simulink library "NCS_Library"  (R2019a)
settings: Solver=VariableStepAuto  StartTime=0.0  StopTime=10.0  RelTol=1e-3
values from neighbouring files (symbols this model uses):
  A = 10    [Parameter.m]
  band = 100000000    [Parameter.m]
  BER = 0    [Parameter.m]
  c = 5000000    [Parameter.m]
  c1 = 4.33    [Parameter.m]
  c2 = 3.16    [Parameter.m]
  CAN2EthernetDelay = 0.000    (= 0)    [Parameter.m]
  cR = 1.5*10^-3    (= 0.0015)    [Parameter.m]
  cw = (cwE * 2 + cwM * (nW_ges-2))/nW_ges    (= 0.1475)    [Parameter.m]
  cwE = 0.35    [Parameter.m]
  cwM = 0.08    [Parameter.m]
  Cycle_Controller = 0    [Parameter.m]
  CyclePLC = 24/1000    (= 0.024)    [Parameter.m]
  d = 800000    [Parameter.m]
  Dr = 0.92    [Parameter.m]
  Ethernet2CANDelay = 0.005    [Parameter.m]
  F_konst = 70892    [Parameter.m]
  FA = 100000    [Parameter.m]
  FB_WB_max = 10000    [Parameter.m]
  FBel_an = iG*nG*F_KZmax*nBan*R_mR/(Dr/2)    (= 28197.4297239)    [Parameter.m]
  FBel_frei = iG*nG*F_KZmax*nBfrei*R_mW/(Dr/2)    (= 29270.6882948)    [Parameter.m]
  Fmaxdyn = 300000    [Parameter.m]
  g = 9.81    [Parameter.m]
  i = 0    [Parameter.m]
  J = 1/2*mA*(Dr/2)^2    (= 158.7)    [Parameter.m]
  k1 = 0.095    [Parameter.m]
  k2 = 9.26/3.6    (= 2.57222222222)    [Parameter.m]
  k3 = 4.63/3.6    (= 1.28611111111)    [Parameter.m]
  mges = 58000    [Parameter.m]
  mu = [mu1 mu2]    [Parameter.m]
  muBel1 = 0.42    [Parameter.m]
  muBel2 = 0.36    [Parameter.m]
  n = 0.001    [Parameter.m]
  n_Mg = 4    [Parameter.m]
  n_WB = 4    [Parameter.m]
  nA = 4    [Parameter.m]
  nBan = 2    [Parameter.m]
  nBfrei = 3    [Parameter.m]
  nM = 4    [Parameter.m]
  nW_an = 4    [Parameter.m]
  P_max = 8200000    [Parameter.m]
  Q = 10    [Parameter.m]
  r_reib = 600    [Parameter.m]
  rho = 1.08    [Parameter.m]
  rhoL = 1.225    [Parameter.m]
  Size = 8    [Parameter.m]
  slip = [s1 s2]    [Parameter.m]
  tol = 0.05    [Parameter.m]
  v00 = 100/3.6    (= 27.7777777778)    [Parameter.m]
  v_grenz = 60/3.6    (= 16.6666666667)    [Parameter.m]
  v_opt = 75/3.6    (= 20.8333333333)    [Parameter.m]
  W_opt = 0.5    [Parameter.m]
  WB = 1    [Parameter.m]
  y_opt = sqrt(W_opt)/((1+sqrt(W_opt))^2+W_opt)    [Parameter.m]
undefined symbols (not defined in the file or in its folder): BUSCapacity, CableLength, controlGate, D_dyn, D_mg, EnableBurst, EnableToF, entity, Entity_out, Gate, Gate_4, Gate_5, Gate_ACK, Gate_copy, Gate_RX, getData, gettime, I_dyn, I_mg, m, magnitude, P_dyn, P_mg, ReadAttributes, readdata, ReadData, ReadSize, sigbuilder_block, Timeout, ToB, ToF, v0, v_d, v_soll
libraries: simulink x176, $bdroot x102
(part 3 of 12)

== system NCS_Library/Plant (Train)/freier Wagen ==
  F_t : Inport
  F_vorne : Inport  Port=2
  F_hinten : Inport  Port=3
  fSt_WB : Inport  Port=4
  Add : Sum  Inputs=+-+--
  Bremskraft Schienenbremse : Subsystem
  Constant : Constant  Value=i
  Display : Display
  Display1 : Display
  Divide : Product  Inputs=*/
  Fahrwiderstand_Wagen : Subsystem
  Integrator : Integrator  InitialCondition=v0  LimitOutput=on  LowerSaturationLimit=tol  ShowSaturationPort=on
  Integrator1 : Integrator
  Scope : Scope
  Wagenmasse : Constant  Value=mges
  rho : Gain  Gain=rho
  v : Outport
  a : Outport  Port=2
  s : Outport  Port=3
  wires:
  rho/1 -> Divide/2
  Add/1 -> Divide/1
  Integrator1/1 -> s/1  "s"
  Constant/1 -> Fahrwiderstand_Wagen/1(Neigung in Promille)
  Wagenmasse/1 -> rho/1, Fahrwiderstand_Wagen/3(mges)
  F_vorne/1 -> Add/3
  Integrator/1 -> v/1, Bremskraft Schienenbremse/1(v), Fahrwiderstand_Wagen/2(v), Integrator1/1  "v"
  F_hinten/1 -> Add/4
  Divide/1 -> Integrator/1, a/1  "a"
  Integrator/2 -> Scope/1
  fSt_WB/1 -> Bremskraft Schienenbremse/2(fSt WB)
  F_t/1 -> Display/1, Add/1
  Bremskraft Schienenbremse/1(FB_frei) -> Add/2
  Fahrwiderstand_Wagen/1(Fw) -> Display1/1, Add/5

== system NCS_Library/Controller/Cookie/Braking Controller ==
  Fahrstufe : Inport
  Bremsstufe : Inport  Port=2
  Notbremse : Inport  Port=3
  v : Inport  Port=4
  Add : Sum
  Bremsen : Subsystem
  Compare To Constant : simulink/Logic and Bit Operations/Compare To Constant  relop===  const=3.0  OutDataTypeStr=boolean
  Compare To Constant1 : simulink/Logic and Bit Operations/Compare To Constant  relop===  const=4  OutDataTypeStr=boolean
  Constant : Constant  Value=v_soll
  Constant1 : Constant
  Demux : Demux  Outputs=3
  Display : Display
  Display1 : Display
  Leerlauf : Subsystem
  Logical Operator : Logic  Operator=OR  AllPortsSameDT=off  OutDataTypeStr=boolean
  Memory : Memory
  Multiport Switch : MultiPortSwitch  Inputs=4  DiagnosticForDefault=None
  Mux : Mux  Inputs=3
  Notbremsung : Subsystem
  Steuerung : Stateflow chart  TreatAsAtomicUnit=on
  konstante Fahrt : Subsystem
  Status : Outport
  fSt : Outport  Port=2
  wires:
  Compare To Constant1/1 -> Logical Operator/2
  Compare To Constant/1 -> Logical Operator/1
  Logical Operator/1 -> Status/1
  Bremsstufe/1 -> Bremsen/2(Bremsstufe)
  Bremsen/1(ST) -> Multiport Switch/4
  Notbremsung/1(ST) -> Multiport Switch/5
  konstante Fahrt/1(fSt) -> Multiport Switch/3
  Leerlauf/1(ST) -> Multiport Switch/2
  Steuerung/1(status) -> Add/2, Display/1, Compare To Constant1/1, Compare To Constant/1
  Constant1/1 -> Add/1
  Multiport Switch/1 -> Memory/1  "fSt"
  v/1 -> Steuerung/4(v), Bremsen/1(v), konstante Fahrt/1(v), Notbremsung/1(v)
  Notbremse/1 -> Steuerung/2(emerg)
  Fahrstufe/1 -> Display1/1, Steuerung/1(fahrst)
  Constant/1 -> Steuerung/3(v_soll)
  Memory/1 -> Demux/1
  Mux/1 -> fSt/1
  Demux/1 -> Mux/2  "fSt_dyn"
  Demux/2 -> Mux/1  "fSt_pneumatic"
  Demux/3 -> Mux/3  "fSt_WB"
  Add/1 -> Multiport Switch/1

== system NCS_Library/Controller/Logic/Braking Controller ==
  Fahrstufe : Inport
  Bremsstufe : Inport  Port=2
  Notbremse : Inport  Port=3
  v : Inport  Port=4
  Add : Sum
  Bremsen : Subsystem
  Compare To Constant : simulink/Logic and Bit Operations/Compare To Constant  relop===  const=3.0  OutDataTypeStr=boolean
  Compare To Constant1 : simulink/Logic and Bit Operations/Compare To Constant  relop===  const=4  OutDataTypeStr=boolean
  Constant : Constant  Value=v_soll
  Constant1 : Constant
  Demux : Demux  Outputs=3
  Display : Display
  Display1 : Display
  Leerlauf : Subsystem
  Logical Operator : Logic  Operator=OR  AllPortsSameDT=off  OutDataTypeStr=boolean
  Memory : Memory
  Multiport Switch : MultiPortSwitch  Inputs=4  DiagnosticForDefault=None
  Mux : Mux  Inputs=3
  Notbremsung : Subsystem
  Steuerung : Stateflow chart  TreatAsAtomicUnit=on
  konstante Fahrt : Subsystem
  Status : Outport
  fSt : Outport  Port=2
  wires:
  Compare To Constant1/1 -> Logical Operator/2
  Compare To Constant/1 -> Logical Operator/1
  Logical Operator/1 -> Status/1
  Bremsstufe/1 -> Bremsen/2(Bremsstufe)
  Bremsen/1(ST) -> Multiport Switch/4
  Notbremsung/1(ST) -> Multiport Switch/5
  konstante Fahrt/1(fSt) -> Multiport Switch/3
  Leerlauf/1(ST) -> Multiport Switch/2
  Steuerung/1(status) -> Add/2, Display/1, Compare To Constant1/1, Compare To Constant/1
  Constant1/1 -> Add/1
  Multiport Switch/1 -> Memory/1  "fSt"
  v/1 -> Steuerung/4(v), Bremsen/1(v), konstante Fahrt/1(v), Notbremsung/1(v)
  Notbremse/1 -> Steuerung/2(emerg)
  Fahrstufe/1 -> Display1/1, Steuerung/1(fahrst)
  Constant/1 -> Steuerung/3(v_soll)
  Memory/1 -> Demux/1
  Mux/1 -> fSt/1
  Demux/1 -> Mux/2  "fSt_dyn"
  Demux/2 -> Mux/1  "fSt_pneumatic"
  Demux/3 -> Mux/3  "fSt_WB"
  Add/1 -> Multiport Switch/1

== system NCS_Library/Controller/Logic/Subsystem ==
  In1 : Inport
  Clock : Clock
  Subtract : Sum  Inputs=-+
  Subtract1 : Sum  Inputs=+-
  Triggered Subsystem : Subsystem  TreatAsAtomicUnit=on
  Triggered Subsystem1 : Subsystem  TreatAsAtomicUnit=on
  Out1 : Outport
  Out2 : Outport  Port=2
  wires:
  Triggered Subsystem1/1(Out1) -> Subtract/2
  Clock/1 -> Triggered Subsystem1/1(In1), Triggered Subsystem/1(In1), Subtract1/1
  Triggered Subsystem/1(Out1) -> Subtract/1, Subtract1/2
  Subtract1/1 -> Out1/1
  Subtract/1 -> Out2/1
  In1/1 -> Triggered Subsystem1/Trigger, Triggered Subsystem/Trigger

== system NCS_Library/Controller/Logic/Subsystem1 ==
  In1 : Inport
  In2 : Inport  Port=2
  Subtract : Sum  Inputs=-+
  Subtract1 : Sum  Inputs=+-
  Triggered Subsystem : Subsystem  TreatAsAtomicUnit=on
  Triggered Subsystem1 : Subsystem  TreatAsAtomicUnit=on
  Out1 : Outport
  Out2 : Outport  Port=2
  wires:
  Triggered Subsystem1/1(Out1) -> Subtract/2
  In2/1 -> Triggered Subsystem1/1(In1), Triggered Subsystem/1(In1), Subtract1/1
  Triggered Subsystem/1(Out1) -> Subtract/1, Subtract1/2
  Subtract1/1 -> Out1/1
  Subtract/1 -> Out2/1
  In1/1 -> Triggered Subsystem1/Trigger, Triggered Subsystem/Trigger

== system NCS_Library/Controller/Logic with PID/konstante Fahrt ==
  Signal : Inport
  v : Inport  Port=2
  Add : Sum  Inputs=|+-
  Constant : Constant  Value=v_d
  Display : Display
  Display1 : Display
  Gain : Gain  Gain=-1
  Multiply : Product
  Mux2 : Mux  Inputs=3
  PID Controller : simulink/Continuous/PID Controller  Controller=PID  Form=Parallel  TimeDomain=Continuous-time  SampleTime=-1  IntegratorMethod=Forward Euler  FilterMethod=Forward Euler  ControllerParametersSource=internal  P=P_dyn  I=I_dyn  D=D_dyn  UseFilter=on  N=100  TunerSelectOption=Transfer Function Based (PID Tuner App)  InitialConditionSource=internal  InitialConditionForIntegrator=0  InitialConditionForFilter=0  DifferentiatorICPrevScaledInput=0  ExternalReset=none  TrackingMode=off  Kt=1  LimitOutput=on  UpperSaturationLimit=1  LowerSaturationLimit=-1  LinearizeAsGain=on  AntiWindupMode=none  Kb=1  POutMin=[]  POutMax=[]  IOutMin=[]  IOutMax=[]  DOutMin=[]  DOutMax=[]  NOutMin=[]  NOutMax=[]  SumOutMin=[]  SumOutMax=[]  SaturationOutMin=[]  SaturationOutMax=[]  PParamMin=[]  PParamMax=[]  IParamMin=[]  IParamMax=[]  DParamMin=[]  DParamMax=[]  NParamMin=[]  NParamMax=[]  KbParamMin=[]  KbParamMax=[]  KtParamMin=[]  KtParamMax=[]  KbOutMin=[]  KbOutMax=[]  KtOutMin=[]  KtOutMax=[]  IntegratorOutMin=[]  IntegratorOutMax=[]  FilterOutMin=[]  FilterOutMax=[]  SumI1OutMin=[]  SumI1OutMax=[]  SumI2OutMin=[]  SumI2OutMax=[]  SumI3OutMin=[]  SumI3OutMax=[]  SumI4OutMin=[]  SumI4OutMax=[]  SumDOutMin=[]  SumDOutMax=[]  DifferentiatorOutMin=[]  DifferentiatorOutMax=[]  FilterDiffOutCoefMin=[]  FilterDiffOutCoefMax=[]  ReciprocalOutMin=[]  ReciprocalOutMax=[]  SumDenOutMin=[]  SumDenOutMax=[]  SumNumOutMin=[]  SumNumOutMax=[]  DivideOutMin=[]  DivideOutMax=[]  IntegratorContinuousStateAttributes=''  IntegratorStateMustResolveToSignalObject=off  IntegratorRTWStateStorageClass=Auto  FilterContinuousStateAttributes=''  FilterStateMustResolveToSignalObject=off  FilterRTWStateStorageClass=Auto  ParallelPVariant=InternalParameters  IdealPVariant=Disabled  IVariant=InternalParameters  DVariant=InternalParameters  IntegratorVariant=Continuous  SatVariant=Enabled  AWVariant=Passthrough  PCopyVariant=Disabled  TRVariant=Disabled  FdbkBlocksVariant=Forward  IdealPFdbkVariant=Disabled  SatFdbkVariant=Disabled  DerivativeFilterVariant=ContFilter  NVariant=InternalParameters  NCopyVariant=Disabled  FilterICVariant=InternalICsFilter  IntegratorICVariant=InternalICs  ExternalResetVariant=Disabled  TRSumVariant=Passthrough  SumFdbkVariant=Disabled  SumVariant=Sum_PID
  PID Controller1 : simulink/Continuous/PID Controller  Controller=PID  Form=Parallel  TimeDomain=Continuous-time  SampleTime=-1  IntegratorMethod=Forward Euler  FilterMethod=Forward Euler  ControllerParametersSource=internal  P=P_mg  I=I_mg  D=D_mg  UseFilter=on  N=100  TunerSelectOption=Transfer Function Based (PID Tuner App)  InitialConditionSource=internal  InitialConditionForIntegrator=0  InitialConditionForFilter=0  DifferentiatorICPrevScaledInput=0  ExternalReset=none  TrackingMode=off  Kt=1  LimitOutput=on  UpperSaturationLimit=1  LowerSaturationLimit=0  LinearizeAsGain=on  AntiWindupMode=none  Kb=1  POutMin=[]  POutMax=[]  IOutMin=[]  IOutMax=[]  DOutMin=[]  DOutMax=[]  NOutMin=[]  NOutMax=[]  SumOutMin=[]  SumOutMax=[]  SaturationOutMin=[]  SaturationOutMax=[]  PParamMin=[]  PParamMax=[]  IParamMin=[]  IParamMax=[]  DParamMin=[]  DParamMax=[]  NParamMin=[]  NParamMax=[]  KbParamMin=[]  KbParamMax=[]  KtParamMin=[]  KtParamMax=[]  KbOutMin=[]  KbOutMax=[]  KtOutMin=[]  KtOutMax=[]  IntegratorOutMin=[]  IntegratorOutMax=[]  FilterOutMin=[]  FilterOutMax=[]  SumI1OutMin=[]  SumI1OutMax=[]  SumI2OutMin=[]  SumI2OutMax=[]  SumI3OutMin=[]  SumI3OutMax=[]  SumI4OutMin=[]  SumI4OutMax=[]  SumDOutMin=[]  SumDOutMax=[]  DifferentiatorOutMin=[]  DifferentiatorOutMax=[]  FilterDiffOutCoefMin=[]  FilterDiffOutCoefMax=[]  ReciprocalOutMin=[]  ReciprocalOutMax=[]  SumDenOutMin=[]  SumDenOutMax=[]  SumNumOutMin=[]  SumNumOutMax=[]  DivideOutMin=[]  DivideOutMax=[]  IntegratorContinuousStateAttributes=''  IntegratorStateMustResolveToSignalObject=off  IntegratorRTWStateStorageClass=Auto  FilterContinuousStateAttributes=''  FilterStateMustResolveToSignalObject=off  FilterRTWStateStorageClass=Auto  ParallelPVariant=InternalParameters  IdealPVariant=Disabled  IVariant=InternalParameters  DVariant=InternalParameters  IntegratorVariant=Continuous  SatVariant=Enabled  AWVariant=Passthrough  PCopyVariant=Disabled  TRVariant=Disabled  FdbkBlocksVariant=Forward  IdealPFdbkVariant=Disabled  SatFdbkVariant=Disabled  DerivativeFilterVariant=ContFilter  NVariant=InternalParameters  NCopyVariant=Disabled  FilterICVariant=InternalICsFilter  IntegratorICVariant=InternalICs  ExternalResetVariant=Disabled  TRSumVariant=Passthrough  SumFdbkVariant=Disabled  SumVariant=Sum_PID
  fSt1 : Constant  Value=0
  f_St : Outport
  wires:
  PID Controller1/1 -> Mux2/3  "f_St,mg"
  PID Controller/1 -> Mux2/1, Display1/1  "f_St,dyn"
  Mux2/1 -> f_St/1
  fSt1/1 -> Mux2/2  "f_St,pneumatic"
  Constant/1 -> Multiply/2
  v/1 -> Add/2  "y_m"
  Add/1 -> Display/1, Gain/1  "e"
  Gain/1 -> PID Controller1/1, PID Controller/1
  Multiply/1 -> Add/1  "w"
  Signal/1 -> Multiply/1

== system NCS_Library/Controller/Subsystem/Signal Builder ==
  Demux : Demux  Tag=STV Demux  Outputs=3
  FromWs : FromWorkspace  Tag=STV FromWs  VariableName=tuvar  SampleTime=0
      SigBuilderData=|
      | common.afterFinalStr = 'Extrapolate'
      | common.sampleTime = 0
      | dataSet.timeRange = [0 200]
      | dataSet.name = 'Group 1'
      | sbobj.Groups.Name = 'Group 1'
      | sbobj.Groups.Signals(1).Name = 'Constant'
      | sbobj.Groups.Signals(1).XData = [0 200]
      | sbobj.Groups.Signals(1).YData = [1 1]
      | sbobj.Groups.Signals(2).Name = 'Arrival'
      | sbobj.Groups.Signals(2).XData = [0 40 40 160 160 200]
      | sbobj.Groups.Signals(2).YData = [1 1 0.0666666666667 0.0666666666667 0.0006 0.0006]
      | sbobj.Groups.Signals(3).Name = 'Notbremsung'
      | sbobj.Groups.Signals(3).XData = [0 60 60 200]
      | sbobj.Groups.Signals(3).YData = [1 1 0 0]
      | sbobj.Groups.TimeRange = [0 200]
  Constant : Outport  Tag=STV Outport
  Arrival : Outport  Tag=STV Outport  Port=2
  Notbremsung : Outport  Tag=STV Outport  Port=3
  wires:
  FromWs/1 -> Demux/1
  Demux/1 -> Constant/1
  Demux/2 -> Arrival/1
  Demux/3 -> Notbremsung/1

== system NCS_Library/Controller/Subsystem1/Signal Builder ==
  Demux : Demux  Tag=STV Demux  Outputs=3
  FromWs : FromWorkspace  Tag=STV FromWs  VariableName=tuvar  SampleTime=0
      SigBuilderData=|
      | common.afterFinalStr = 'Extrapolate'
      | common.sampleTime = 0
      | dataSet.timeRange = [0 200]
      | dataSet.name = 'Group 1'
      | sbobj.Groups.Name = 'Group 1'
      | sbobj.Groups.Signals(1).Name = 'Konstante Fahrt'
      | sbobj.Groups.Signals(1).XData = [0 200]
      | sbobj.Groups.Signals(1).YData = [1 1]
      | sbobj.Groups.Signals(2).Name = 'Betriebsbremsung'
      | sbobj.Groups.Signals(2).XData = [0 20 20 160 160 200]
      | sbobj.Groups.Signals(2).YData = [1 1 0.2 0.2 1 1]
      | sbobj.Groups.Signals(3).Name = 'Notbremsung'
      | sbobj.Groups.Signals(3).XData = [0 60 60 200]
      | sbobj.Groups.Signals(3).YData = [1 1 0 0]
      | sbobj.Groups.TimeRange = [0 200]
  Konstante Fahrt : Outport  Tag=STV Outport
  Betriebsbremsung : Outport  Tag=STV Outport  Port=2
  Notbremsung : Outport  Tag=STV Outport  Port=3
  wires:
  Demux/3 -> Notbremsung/1
  Demux/2 -> Betriebsbremsung/1
  Demux/1 -> Konstante Fahrt/1
  FromWs/1 -> Demux/1

== system NCS_Library/Network/Applications/Failure Control ==
  In : Inport
  Add : Sum  Inputs=+++
  Clock : Clock
  Compare To Constant : simulink/Logic and Bit Operations/Compare To Constant  relop=>=  const=ToF  OutDataTypeStr=uint8
  Compare To Zero : simulink/Logic and Bit Operations/Compare To Zero  relop=>  OutDataTypeStr=uint8
  Constant : Constant  Value=EnableToF
  Constant1 : Constant  OutDataTypeStr=uint8
  Display : Display
  Display1 : Display
  Entity Input Switch : EntityInputSwitch  InputPortMessageModes=m,m  OutputPortMessageModes=m
  Entity Output Switch : EntityOutputSwitch  InputPortMessageModes=m,m  OutputPortMessageModes=m,m,m  NumberOutputPorts=3  SwitchingCriterion=From control port  SwitchAttributeName=Attribute1
      settings: InputPortMap=u0,u1  OutputPortMap=o0,o1,o2
  Entity Server : EntityServer  InputPortMessageModes=m  OutputPortMessageModes=n,m  Capacity=1  ServiceTimeValue=0  EntryAction=entity.Data = DeleteData();  NumberEntitiesDeparted=on
      settings: OutputPortMap=o0,o9
  Entity Terminator : EntityTerminator  InputPortMessageModes=m
  Logical Operator : Logic  AllPortsSameDT=off  OutDataTypeStr=boolean
  Message Send : MessageSend  OutputPortMessageModes=m
      settings: InputPortMap=u1
  Simulink Function : Subsystem  TreatAsAtomicUnit=on
  Out : Outport
  wires:
  Entity Output Switch/1 -> Entity Input Switch/1  "Device OK"
  In/1 -> Entity Output Switch/2
  Entity Output Switch/3 -> Entity Terminator/1  "Failure"
  Clock/1 -> Compare To Constant/1
  Compare To Constant/1 -> Display1/1, Logical Operator/1
  Constant/1 -> Display/1, Logical Operator/2
  Message Send/1 -> Entity Output Switch/1
  Logical Operator/1 -> Add/1
  Add/1 -> Message Send/1
  Constant1/1 -> Add/2
  Entity Output Switch/2 -> Entity Server/1  "Set Data to 0"
  Entity Input Switch/1 -> Out/1
  Entity Server/2 -> Entity Input Switch/2
  Entity Server/1 -> Compare To Zero/1
  Compare To Zero/1 -> Add/3

== system NCS_Library/Network/Applications/Failure Control CAN ==
  In : Inport
  Add : Sum  Inputs=|++
  Clock : Clock
  Compare To Constant : simulink/Logic and Bit Operations/Compare To Constant  relop=>=  const=ToF  OutDataTypeStr=uint8
  Constant : Constant  Value=EnableToF
  Constant1 : Constant  OutDataTypeStr=uint8
  Display : Display
  Display1 : Display
  Entity Output Switch : EntityOutputSwitch  InputPortMessageModes=m,m  OutputPortMessageModes=m,m  SwitchingCriterion=From control port  SwitchAttributeName=Attribute1
      settings: InputPortMap=u0,u1
  Entity Terminator : EntityTerminator  InputPortMessageModes=m
  Logical Operator : Logic  AllPortsSameDT=off  OutDataTypeStr=boolean
  Message Send : MessageSend  OutputPortMessageModes=m
      settings: InputPortMap=u1
  Out : Outport
  wires:
  Constant1/1 -> Add/2
  Add/1 -> Message Send/1
  Logical Operator/1 -> Add/1
  Message Send/1 -> Entity Output Switch/1
  Constant/1 -> Logical Operator/2, Display/1
  Compare To Constant/1 -> Logical Operator/1, Display1/1
  Clock/1 -> Compare To Constant/1
  Entity Output Switch/2 -> Entity Terminator/1  "Failure"
  In/1 -> Entity Output Switch/2
  Entity Output Switch/1 -> Out/1  "Device OK"

== system NCS_Library/Network/Applications/Multiplexer ==
  Demux : MATLAB Function  TreatAsAtomicUnit=on
  Demux CAN : MATLAB Function  TreatAsAtomicUnit=on
  Demux Consist : MATLAB Function  TreatAsAtomicUnit=on
  MUX ECN : MATLAB Function  TreatAsAtomicUnit=on
  Mux : MATLAB Function  TreatAsAtomicUnit=on
  Mux Consist : MATLAB Function  TreatAsAtomicUnit=on
  Mux Reference Y_M : MATLAB Function  TreatAsAtomicUnit=on
  Mux U : MATLAB Function  TreatAsAtomicUnit=on
  Mux y_m : MATLAB Function  TreatAsAtomicUnit=on
  MuxCAN : MATLAB Function  TreatAsAtomicUnit=on

== system NCS_Library/Network/Applications/NetworkSelector ==
  Constant : Constant  Value=NetworkType  OutDataTypeStr=uint8
  Demux : MATLAB Function  TreatAsAtomicUnit=on
  Demux CAN : MATLAB Function  TreatAsAtomicUnit=on
  Demux CAN1 : MATLAB Function  TreatAsAtomicUnit=on
  Demux Consist : MATLAB Function  TreatAsAtomicUnit=on
  Demux1 : MATLAB Function  TreatAsAtomicUnit=on
  Multiport Switch : MultiPortSwitch  Inputs=4
  tag scope: Y_M_1=global, Y_M_2=global, u_1=global, u_2=global, u_3=global, u_4=global, u_5=global, u_6=global, u_7=global, u_8=global
  wires:
  Demux Consist/2(out_2) -> Demux1/1(in)
  Demux Consist/1(out_1) -> Demux/1(in)
  Demux CAN1/4(u4) -> [u_8]
  Demux CAN1/2(u2) -> [u_6]
  Demux CAN/2(u2) -> [u_2]
  Demux1/2(Y_M) -> [Y_M_2]
  Demux CAN/3(u3) -> [u_3]
  Demux/2(Y_M) -> [Y_M_1]
  Demux1/1(U) -> Demux CAN1/1(U)
  Demux CAN1/3(u3) -> [u_7]
  Demux/1(U) -> Demux CAN/1(U)
  Demux CAN/4(u4) -> [u_4]
  Demux CAN/1(u1) -> [u_1]
  Demux CAN1/1(u1) -> [u_5]
  Multiport Switch/1 -> Demux Consist/1(in)
  [Reference] -> Multiport Switch/2
  Constant/1 -> Multiport Switch/1
  [CAN] -> Multiport Switch/3
  [Ethernet] -> Multiport Switch/4
  [EthernetCAN_Ring] -> Multiport Switch/5

== system NCS_Library/Network/Applications/Subsystem ==
  Burst Control : Stateflow chart  TreatAsAtomicUnit=on
  Clock : Clock
  Compare To Constant : simulink/Logic and Bit Operations/Compare To Constant  relop=>=  const=ToB  OutDataTypeStr=uint8
  Constant : Constant  Value=EnableBurst
  Burst : Outport
  wires:
  Constant/1 -> Burst Control/2(Enable)
  Compare To Constant/1 -> Burst Control/1(ToF)
  Clock/1 -> Compare To Constant/1
  Burst Control/1(Burst) -> Burst/1

== system NCS_Library/Network/Applications/TRDP Timeout ==
  #Reveive : Inport
  Chart : Stateflow chart  TreatAsAtomicUnit=on
  Clock : Clock
  Constant : Constant  Value=Timeout
  Detect Change : simulink/Logic and Bit Operations/Detect Change  vinit=0  OutDataTypeStr=boolean
  Display : Display
  Display1 : Display
  Display2 : Display
  Valid : Outport
  wires:
  Chart/1(Valid) -> Valid/1
  #Reveive/1 -> Display/1, Detect Change/1
  Constant/1 -> Chart/1(Timeout)
  Detect Change/1 -> Display1/1, Chart/2(Restart_Timer)
  Clock/1 -> Display2/1, Chart/3(currentTime)

== system NCS_Library/Network/Applications/Watch Dog ==
  Device : Inport
  Constant : Constant  Value=2
  Detect Change : simulink/Logic and Bit Operations/Detect Change  vinit=0  OutDataTypeStr=boolean
  Display : Display
  Timeout Watch Dog : Stateflow chart  TreatAsAtomicUnit=on
  Failed : Outport
  wires:
  Device/1 -> Detect Change/1
  Detect Change/1 -> Display/1, Timeout Watch Dog/1(Msg)
  Constant/1 -> Timeout Watch Dog/2(Timeout)
  Timeout Watch Dog/1(Failed) -> Failed/1

== system NCS_Library/Network/CAN/CAN BUS ==
  note: CAN Bus
  Arbitration on Message Priority : EntityQueue  OutputPortMessageModes=m  QueueType=Priority  PrioritySource=ID  EntityArrivalSource=Multicast  MulticastTag=ToBus_1
      settings: OutputPortMap=o5
  Broadcast to Receivers : EntityMulticast  InputPortMessageModes=m  MulticastTag=FromBus_1
  Communication Delay : EntityServer  InputPortMessageModes=m  OutputPortMessageModes=n,m  Capacity=1  ServiceTimeSource=Attribute  ServiceTimeAttributeName=CommDelay  EntryAction=controlGate(0);  ServiceCompleteAction=entity.RndLoss = setLossState();  ExitAction=controlGate(1);  SortingAttributeName=ID  Utilization=on
      settings: OutputPortMap=o5,o9
  Drop Low Priority Messages : EntityTerminator  InputPortMessageModes=m
  Enable Gate : EntityGate  InputPortMessageModes=m,m  OutputPortMessageModes=m  OpenGateAtSimulationStart=on
  Entity Output Switch : EntityOutputSwitch  InputPortMessageModes=m  OutputPortMessageModes=m,m  SwitchAttributeName=Attribute1
  Goto : Goto  Commented=on  GotoTag=util  TagVisibility=global
  Simulink Function : Subsystem  TreatAsAtomicUnit=on
  Simulink Function1 : Subsystem  TreatAsAtomicUnit=on
  wires:
  Communication Delay/1 -> Goto/1
  Enable Gate/1 -> Communication Delay/1
  Simulink Function1/1(ctrl) -> Enable Gate/1
  Communication Delay/2 -> Broadcast to Receivers/1
  Arbitration on Message Priority/1 -> Entity Output Switch/1
  Entity Output Switch/2 -> Drop Low Priority Messages/1
  Entity Output Switch/1 -> Enable Gate/2

== system NCS_Library/Network/CAN/CAN BUS1 ==
  note: CAN Bus
  Arbitration on Message Priority : EntityQueue  OutputPortMessageModes=m  QueueType=Priority  PrioritySource=ID  EntityArrivalSource=Multicast  MulticastTag=ToBus_2
      settings: OutputPortMap=o5
  Broadcast to Receivers : EntityMulticast  InputPortMessageModes=m  MulticastTag=FromBus_2
  Communication Delay : EntityServer  InputPortMessageModes=m  OutputPortMessageModes=n,m  Capacity=1  ServiceTimeSource=Attribute  ServiceTimeAttributeName=CommDelay  EntryAction=controlGate(0);  ServiceCompleteAction=entity.RndLoss = setLossState();  ExitAction=controlGate(1);  SortingAttributeName=ID  Utilization=on
      settings: OutputPortMap=o5,o9
  Drop Low Priority Messages : EntityTerminator  InputPortMessageModes=m
  Enable Gate : EntityGate  InputPortMessageModes=m,m  OutputPortMessageModes=m  OpenGateAtSimulationStart=on
  Entity Output Switch : EntityOutputSwitch  InputPortMessageModes=m  OutputPortMessageModes=m,m  SwitchAttributeName=Attribute1
  Goto : Goto  Commented=on  GotoTag=util  TagVisibility=global
  Simulink Function : Subsystem  TreatAsAtomicUnit=on
  Simulink Function1 : Subsystem  TreatAsAtomicUnit=on
  wires:
  Entity Output Switch/1 -> Enable Gate/2
  Entity Output Switch/2 -> Drop Low Priority Messages/1
  Arbitration on Message Priority/1 -> Entity Output Switch/1
  Communication Delay/2 -> Broadcast to Receivers/1
  Simulink Function1/1(ctrl) -> Enable Gate/1
  Enable Gate/1 -> Communication Delay/1
  Communication Delay/1 -> Goto/1

== system NCS_Library/Network/CAN/CAN Node 1 ==
  note: Receiver
  note: Transmitter
  d_in : Inport
  Compare To Constant : simulink/Logic and Bit Operations/Compare To Constant  relop=<=  const=3.0  OutDataTypeStr=boolean
  Constant : Constant  Value=SensorType
  Current Message : EntityQueue  InputPortMessageModes=m  OutputPortMessageModes=m  Capacity=2  EntryAction=controlGate(0);  ExitAction=controlGate(1);
      settings: OutputPortMap=o5
  Damaged Message : EntityTerminator  InputPortMessageModes=m  NumberEntitiesArrived=on
      settings: OutputPortMap=o0
  Display{,1..4} (5 alike) : Display
  Drop Dated Message upon Buffer Overflow : EntityOutputSwitch  InputPortMessageModes=m  OutputPortMessageModes=m,m  SwitchAttributeName=Attribute1
  Entity Replicator : EntityReplicator  InputPortMessageModes=m  OutputPortMessageModes=m,m
  Entity Terminator : EntityTerminator  InputPortMessageModes=m
  Failure Control CAN : $bdroot/Network/Applications/Failure Control CAN  SystemSampleTime=-1
  Failure Control CAN1 : $bdroot/Network/Applications/Failure Control CAN  SystemSampleTime=-1
  Message Release Control : EntityGate  InputPortMessageModes=m,m  OutputPortMessageModes=m  OpenGateAtSimulationStart=on
  Message from Bus : EntityQueue  OutputPortMessageModes=m  Capacity=20  EntityArrivalSource=Multicast  MulticastTag=FromBus_1
      settings: OutputPortMap=o5
  Path Combiner : EntityInputSwitch  InputPortMessageModes=m,m  OutputPortMessageModes=m
  Re-Transmission Control : Subsystem
  Received Message : EntityServer  InputPortMessageModes=m  OutputPortMessageModes=m  Capacity=1  ServiceTimeValue=0
  Reception Control : Stateflow chart  TreatAsAtomicUnit=on
  Replicate for Re-Transmission : EntityReplicator  InputPortMessageModes=m  OutputPortMessageModes=m,m,m  NumberReplicas=2
      settings: OutputPortMap=o0,o1,o2
  Send Message to Bus : EntityMulticast  InputPortMessageModes=m  MulticastTag=ToBus_1
  Signal To CAN Message : Subsystem
  Simulink Function : Subsystem  TreatAsAtomicUnit=on
  Simulink Function1 : Subsystem  TreatAsAtomicUnit=on
  Sort : EntityOutputSwitch  InputPortMessageModes=m,m  OutputPortMessageModes=m,m,m  NumberOutputPorts=3  SwitchingCriterion=From control port  SwitchAttributeName=Attribute1
      settings: InputPortMap=u0,u1  OutputPortMap=o0,o1,o2
  Subscribed Message : EntityTerminator  InputPortMessageModes=m  EntryAction=getData(entity.Data, entity.f_St);  NumberEntitiesArrived=on
      settings: OutputPortMap=o0
  Switch : Switch  Criteria=u2 > Threshold
  Transmission Buffer : EntityQueue  InputPortMessageModes=m  OutputPortMessageModes=m  Capacity=15  QueueType=Priority  PrioritySource=ID
      settings: OutputPortMap=o5
  Unsubscribed Message : EntityTerminator  InputPortMessageModes=m  NumberEntitiesArrived=on
      settings: OutputPortMap=o0
  d_out : Outport
  wires:
  Reception Control/3(ReTX) -> [ReTX]
  Re-Transmission Control/2(#TX) -> Display3/1
  d_in/1 -> Signal To CAN Message/1(Data)
  [ReTX] -> Re-Transmission Control/2(ReTX)
  Received Message/1 -> Sort/2
  Path Combiner/1 -> Transmission Buffer/1
  Message Release Control/1 -> Replicate for Re-Transmission/1
  Replicate for Re-Transmission/1 -> Current Message/1
  Message from Bus/1 -> Failure Control CAN/1
  [Reset] -> Re-Transmission Control/3(Reset)
  Sort/2 -> Unsubscribed Message/1
  Sort/3 -> Damaged Message/1
  Sort/1 -> Subscribed Message/1
  Entity Replicator/2 -> Received Message/1
  Entity Replicator/1 -> Reception Control/2(RX)
  Reception Control/2(Success) -> [Reset]
  Reception Control/1(Port) -> Sort/1
  Simulink Function1/1(data) -> Switch/1
  Current Message/1 -> Re-Transmission Control/1(IN)
  Replicate for Re-Transmission/3 -> Reception Control/1(TX)
  Simulink Function/1(ctrl) -> Message Release Control/1
  Replicate for Re-Transmission/2 -> Send Message to Bus/1
  Drop Dated Message upon Buffer Overflow/1 -> Path Combiner/1
  Drop Dated Message upon Buffer Overflow/2 -> Entity Terminator/1
  Damaged Message/1 -> Display/1
  Unsubscribed Message/1 -> Display1/1
  Subscribed Message/1 -> Display2/1
  Signal To CAN Message/1(MsgOut) -> Path Combiner/2
  Failure Control CAN/1 -> Entity Replicator/1
  Re-Transmission Control/1(OUT) -> Drop Dated Message upon Buffer Overflow/1
  Transmission Buffer/1 -> Failure Control CAN1/1
  Failure Control CAN1/1 -> Message Release Control/2
  Simulink Function1/2(f_St) -> Switch/3
  Switch/1 -> Display4/1, d_out/1
  Constant/1 -> Compare To Constant/1
  Compare To Constant/1 -> Switch/2

== system NCS_Library/Network/CAN/CAN Node 2 ==
  note: Transmitter
  note: Receiver
  d_in : Inport
  Compare To Constant : simulink/Logic and Bit Operations/Compare To Constant  relop=<=  const=3.0  OutDataTypeStr=boolean
  Constant : Constant  Value=SensorType
  Current Message : EntityQueue  InputPortMessageModes=m  OutputPortMessageModes=m  Capacity=2  EntryAction=controlGate(0);  ExitAction=controlGate(1);
      settings: OutputPortMap=o5
  Damaged Message : EntityTerminator  InputPortMessageModes=m  NumberEntitiesArrived=on
      settings: OutputPortMap=o0
  Display{,1..4} (5 alike) : Display
  Drop Dated Message upon Buffer Overflow : EntityOutputSwitch  InputPortMessageModes=m  OutputPortMessageModes=m,m  SwitchAttributeName=Attribute1
  Entity Replicator : EntityReplicator  InputPortMessageModes=m  OutputPortMessageModes=m,m
  Entity Terminator : EntityTerminator  InputPortMessageModes=m
  Failure Control CAN : $bdroot/Network/Applications/Failure Control CAN  SystemSampleTime=-1
  Failure Control CAN1 : $bdroot/Network/Applications/Failure Control CAN  SystemSampleTime=-1
  Message Release Control : EntityGate  InputPortMessageModes=m,m  OutputPortMessageModes=m  OpenGateAtSimulationStart=on
  Message from Bus : EntityQueue  OutputPortMessageModes=m  Capacity=20  EntityArrivalSource=Multicast  MulticastTag=FromBus_2
      settings: OutputPortMap=o5
  Path Combiner : EntityInputSwitch  InputPortMessageModes=m,m  OutputPortMessageModes=m
  Re-Transmission Control : Subsystem
  Received Message : EntityServer  InputPortMessageModes=m  OutputPortMessageModes=m  Capacity=1  ServiceTimeValue=0
  Reception Control : Stateflow chart  TreatAsAtomicUnit=on
  Replicate for Re-Transmission : EntityReplicator  InputPortMessageModes=m  OutputPortMessageModes=m,m,m  NumberReplicas=2
      settings: OutputPortMap=o0,o1,o2
  Send Message to Bus : EntityMulticast  InputPortMessageModes=m  MulticastTag=ToBus_2
  Signal To CAN Message : Subsystem
  Simulink Function : Subsystem  TreatAsAtomicUnit=on
  Simulink Function1 : Subsystem  TreatAsAtomicUnit=on
  Sort : EntityOutputSwitch  InputPortMessageModes=m,m  OutputPortMessageModes=m,m,m  NumberOutputPorts=3  SwitchingCriterion=From control port  SwitchAttributeName=Attribute1
      settings: InputPortMap=u0,u1  OutputPortMap=o0,o1,o2
  Subscribed Message : EntityTerminator  InputPortMessageModes=m  EntryAction=getData(entity.Data, entity.f_St);  NumberEntitiesArrived=on
      settings: OutputPortMap=o0
  Switch : Switch  Criteria=u2 > Threshold
  Transmission Buffer : EntityQueue  InputPortMessageModes=m  OutputPortMessageModes=m  Capacity=15  QueueType=Priority  PrioritySource=ID
      settings: OutputPortMap=o5
  Unsubscribed Message : EntityTerminator  InputPortMessageModes=m  NumberEntitiesArrived=on
      settings: OutputPortMap=o0
  d_out : Outport
  wires:
  Compare To Constant/1 -> Switch/2
  Constant/1 -> Compare To Constant/1
  Switch/1 -> d_out/1, Display4/1
  Simulink Function1/2(f_St) -> Switch/3
  Failure Control CAN/1 -> Message Release Control/2
  Transmission Buffer/1 -> Failure Control CAN/1
  Re-Transmission Control/1(OUT) -> Drop Dated Message upon Buffer Overflow/1
  Failure Control CAN1/1 -> Entity Replicator/1
  Signal To CAN Message/1(MsgOut) -> Path Combiner/2
  Subscribed Message/1 -> Display2/1
  Unsubscribed Message/1 -> Display1/1
  Damaged Message/1 -> Display/1
  Drop Dated Message upon Buffer Overflow/2 -> Entity Terminator/1
  Drop Dated Message upon Buffer Overflow/1 -> Path Combiner/1
  Replicate for Re-Transmission/2 -> Send Message to Bus/1
  Simulink Function/1(ctrl) -> Message Release Control/1
  Replicate for Re-Transmission/3 -> Reception Control/1(TX)
  Current Message/1 -> Re-Transmission Control/1(IN)
  Simulink Function1/1(data) -> Switch/1
  Reception Control/1(Port) -> Sort/1
  Reception Control/2(Success) -> [Reset]
  Entity Replicator/1 -> Reception Control/2(RX)
  Entity Replicator/2 -> Received Message/1
  Sort/1 -> Subscribed Message/1
  Sort/3 -> Damaged Message/1
  Sort/2 -> Unsubscribed Message/1
  [Reset] -> Re-Transmission Control/3(Reset)
  Message from Bus/1 -> Failure Control CAN1/1
  Replicate for Re-Transmission/1 -> Current Message/1
  Message Release Control/1 -> Replicate for Re-Transmission/1
  Path Combiner/1 -> Transmission Buffer/1
  Received Message/1 -> Sort/2
  [ReTX] -> Re-Transmission Control/2(ReTX)
  d_in/1 -> Signal To CAN Message/1(Data)
  Re-Transmission Control/2(#TX) -> Display3/1
  Reception Control/3(ReTX) -> [ReTX]

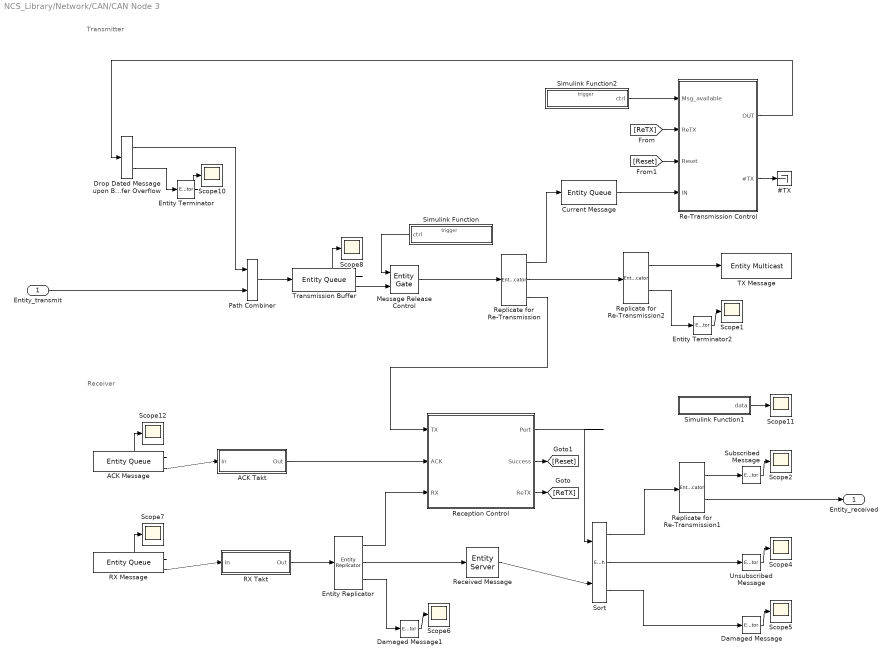
== system NCS_Library/Network/CAN/CAN Node 3 ==
  note: Transmitter
  note: Receiver
  Entity_transmit : Inport
  #TX : Terminator
  ACK Message : EntityQueue  OutputPortMessageModes=n,m  Capacity=20  EntityArrivalSource=Multicast  MulticastTag=FromBus_1  NumberEntitiesInBlock=on
      settings: OutputPortMap=o1,o5
  ACK Takt : Subsystem
  Current Message : EntityQueue  InputPortMessageModes=m  OutputPortMessageModes=m  Capacity=2  EntryAction=|  ExitAction=|
      EntryAction=|
      | Gate_TX(0);
      | Msg_available(1);
      ExitAction=|
      | Gate_TX(1);
      | Msg_available(0);
      settings: OutputPortMap=o5
  Damaged Message : EntityTerminator  InputPortMessageModes=m  NumberEntitiesArrived=on
      settings: OutputPortMap=o0
  Damaged Message1 : EntityTerminator  InputPortMessageModes=m  NumberEntitiesArrived=on
      settings: OutputPortMap=o0
  Drop Dated Message upon Buffer Overflow : EntityOutputSwitch  InputPortMessageModes=m  OutputPortMessageModes=m,m  SwitchAttributeName=Attribute1
  Entity Replicator : EntityReplicator  InputPortMessageModes=m  OutputPortMessageModes=m,m,m  NumberReplicas=2
      settings: OutputPortMap=o0,o1,o2
  Entity Terminator : EntityTerminator  InputPortMessageModes=m  NumberEntitiesArrived=on
      settings: OutputPortMap=o0
  Entity Terminator2 : EntityTerminator  InputPortMessageModes=m  NumberEntitiesArrived=on
      settings: OutputPortMap=o0
  Message Release Control : EntityGate  InputPortMessageModes=m,m  OutputPortMessageModes=m  OpenGateAtSimulationStart=on
  Path Combiner : EntityInputSwitch  InputPortMessageModes=m,m  OutputPortMessageModes=m
  RX Message : EntityQueue  OutputPortMessageModes=n,m  Capacity=20  EntityArrivalSource=Multicast  MulticastTag=FromBus_2  NumberEntitiesInBlock=on
      settings: OutputPortMap=o1,o5
  RX Takt : Subsystem
  Re-Transmission Control : Subsystem
  Received Message : EntityServer  InputPortMessageModes=m  OutputPortMessageModes=m  Capacity=1  ServiceTimeValue=0
  Reception Control : Stateflow chart  TreatAsAtomicUnit=on
  Replicate for Re-Transmission : EntityReplicator  InputPortMessageModes=m  OutputPortMessageModes=m,m,m  NumberReplicas=2
      settings: OutputPortMap=o0,o1,o2
  Replicate for Re-Transmission1 : EntityReplicator  InputPortMessageModes=m  OutputPortMessageModes=m,m
  Replicate for Re-Transmission2 : EntityReplicator  InputPortMessageModes=m  OutputPortMessageModes=m,m
  Scope{1..2,4..8,10..12} (10 alike) : Scope
  Simulink Function : Subsystem  TreatAsAtomicUnit=on
  Simulink Function1 : Subsystem  TreatAsAtomicUnit=on
  Simulink Function2 : Subsystem  TreatAsAtomicUnit=on
  Sort : EntityOutputSwitch  InputPortMessageModes=m,m  OutputPortMessageModes=m,m,m  NumberOutputPorts=3  SwitchingCriterion=From control port  SwitchAttributeName=Attribute1
      settings: InputPortMap=u0,u1  OutputPortMap=o0,o1,o2
  Subscribed Message : EntityTerminator  InputPortMessageModes=m  EntryAction=|  NumberEntitiesArrived=on
      | getData(entity.Data);
      | %calcDelay(entity.Time);
      settings: OutputPortMap=o0
  TX Message : EntityMulticast  InputPortMessageModes=m  MulticastTag=ToBus_1
  Transmission Buffer : EntityQueue  InputPortMessageModes=m  OutputPortMessageModes=n,m  Capacity=15  QueueType=Priority  PrioritySource=ID  NumberEntitiesInBlock=on
      settings: OutputPortMap=o1,o5
  Unsubscribed Message : EntityTerminator  InputPortMessageModes=m  NumberEntitiesArrived=on
      settings: OutputPortMap=o0
  Entity_received : Outport
  wires:
  RX Message/2 -> RX Takt/1(In)
  ACK Message/2 -> ACK Takt/1(In)
  ACK Takt/1(Out) -> Reception Control/2(ACK)
  Transmission Buffer/1 -> Scope8/1
  Damaged Message/1 -> Scope5/1
  Unsubscribed Message/1 -> Scope4/1
  Re-Transmission Control/1(OUT) -> Drop Dated Message upon Buffer Overflow/1
  Replicate for Re-Transmission/2 -> Replicate for Re-Transmission2/1
  Simulink Function/1(ctrl) -> Message Release Control/1
  Replicate for Re-Transmission/3 -> Reception Control/1(TX)
  Reception Control/1(Port) -> Sort/1
  Reception Control/2(Success) -> [Reset]
  Entity Replicator/2 -> Received Message/1
  Sort/3 -> Damaged Message/1
  Sort/2 -> Unsubscribed Message/1
  [Reset] -> Re-Transmission Control/3(Reset)
  Replicate for Re-Transmission/1 -> Current Message/1
  Message Release Control/1 -> Replicate for Re-Transmission/1
  Transmission Buffer/2 -> Message Release Control/2
  Received Message/1 -> Sort/2
  [ReTX] -> Re-Transmission Control/2(ReTX)
  Reception Control/3(ReTX) -> [ReTX]
  Damaged Message1/1 -> Scope6/1
  Entity Replicator/3 -> Damaged Message1/1
  Entity Terminator2/1 -> Scope1/1
  Current Message/1 -> Re-Transmission Control/4(IN)
  Drop Dated Message upon Buffer Overflow/1 -> Path Combiner/1
  Re-Transmission Control/2(#TX) -> #TX/1
  RX Message/1 -> Scope7/1
  Sort/1 -> Replicate for Re-Transmission1/1
  Entity_transmit/1 -> Path Combiner/2
  Entity Replicator/1 -> Reception Control/3(RX)
  ACK Message/1 -> Scope12/1
  Entity Terminator/1 -> Scope10/1
  Simulink Function2/1(ctrl) -> Re-Transmission Control/1(Msg_available)
  Drop Dated Message upon Buffer Overflow/2 -> Entity Terminator/1
  Path Combiner/1 -> Transmission Buffer/1
  RX Takt/1(Out) -> Entity Replicator/1
  Simulink Function1/1(data) -> Scope11/1
  Replicate for Re-Transmission2/1 -> TX Message/1
  Replicate for Re-Transmission2/2 -> Entity Terminator2/1
  Subscribed Message/1 -> Scope2/1
  Replicate for Re-Transmission1/2 -> Entity_received/1
  Replicate for Re-Transmission1/1 -> Subscribed Message/1

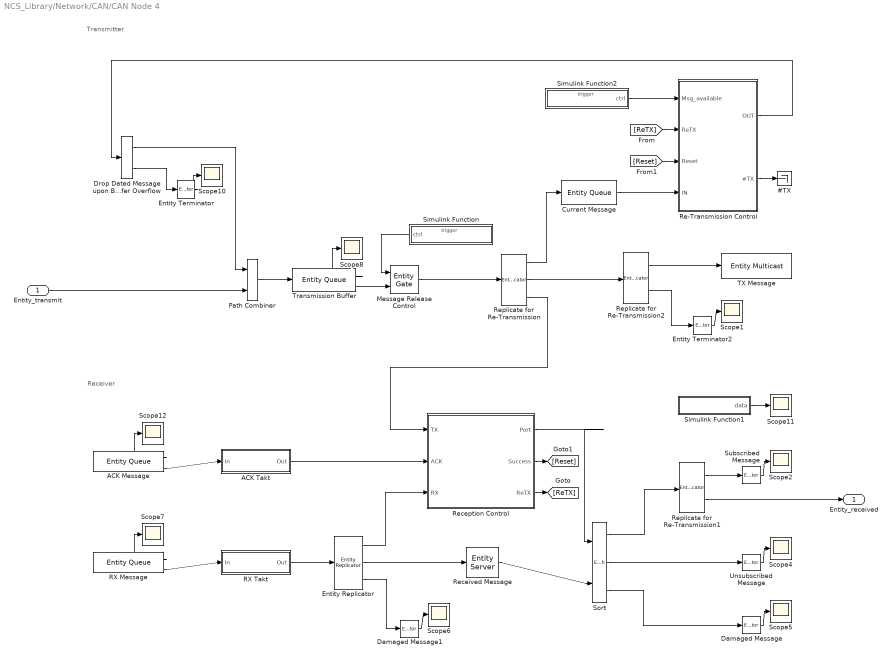
== system NCS_Library/Network/CAN/CAN Node 4 ==
  note: Receiver
  note: Transmitter
  Entity_transmit : Inport
  #TX : Terminator
  ACK Message : EntityQueue  OutputPortMessageModes=n,m  Capacity=20  EntityArrivalSource=Multicast  MulticastTag=FromBus_2  NumberEntitiesInBlock=on
      settings: OutputPortMap=o1,o5
  ACK Takt : Subsystem
  Current Message : EntityQueue  InputPortMessageModes=m  OutputPortMessageModes=m  Capacity=2  EntryAction=|  ExitAction=|
      EntryAction=|
      | Gate_TX(0);
      | Msg_available(1);
      ExitAction=|
      | Gate_TX(1);
      | Msg_available(0);
      settings: OutputPortMap=o5
  Damaged Message : EntityTerminator  InputPortMessageModes=m  NumberEntitiesArrived=on
      settings: OutputPortMap=o0
  Damaged Message1 : EntityTerminator  InputPortMessageModes=m  NumberEntitiesArrived=on
      settings: OutputPortMap=o0
  Drop Dated Message upon Buffer Overflow : EntityOutputSwitch  InputPortMessageModes=m  OutputPortMessageModes=m,m  SwitchAttributeName=Attribute1
  Entity Replicator : EntityReplicator  InputPortMessageModes=m  OutputPortMessageModes=m,m,m  NumberReplicas=2
      settings: OutputPortMap=o0,o1,o2
  Entity Terminator : EntityTerminator  InputPortMessageModes=m  NumberEntitiesArrived=on
      settings: OutputPortMap=o0
  Entity Terminator2 : EntityTerminator  InputPortMessageModes=m  NumberEntitiesArrived=on
      settings: OutputPortMap=o0
  Message Release Control : EntityGate  InputPortMessageModes=m,m  OutputPortMessageModes=m  OpenGateAtSimulationStart=on
  Path Combiner : EntityInputSwitch  InputPortMessageModes=m,m  OutputPortMessageModes=m
  RX Message : EntityQueue  OutputPortMessageModes=n,m  Capacity=20  EntityArrivalSource=Multicast  MulticastTag=FromBus_1  NumberEntitiesInBlock=on
      settings: OutputPortMap=o1,o5
  RX Takt : Subsystem
  Re-Transmission Control : Subsystem
  Received Message : EntityServer  InputPortMessageModes=m  OutputPortMessageModes=m  Capacity=1  ServiceTimeValue=0
  Reception Control : Stateflow chart  TreatAsAtomicUnit=on
  Replicate for Re-Transmission : EntityReplicator  InputPortMessageModes=m  OutputPortMessageModes=m,m,m  NumberReplicas=2
      settings: OutputPortMap=o0,o1,o2
  Replicate for Re-Transmission1 : EntityReplicator  InputPortMessageModes=m  OutputPortMessageModes=m,m
  Replicate for Re-Transmission2 : EntityReplicator  InputPortMessageModes=m  OutputPortMessageModes=m,m
  Scope{1..2,4..8,10..12} (10 alike) : Scope
  Simulink Function : Subsystem  TreatAsAtomicUnit=on
  Simulink Function1 : Subsystem  TreatAsAtomicUnit=on
  Simulink Function2 : Subsystem  TreatAsAtomicUnit=on
  Sort : EntityOutputSwitch  InputPortMessageModes=m,m  OutputPortMessageModes=m,m,m  NumberOutputPorts=3  SwitchingCriterion=From control port  SwitchAttributeName=Attribute1
      settings: InputPortMap=u0,u1  OutputPortMap=o0,o1,o2
  Subscribed Message : EntityTerminator  InputPortMessageModes=m  EntryAction=|  NumberEntitiesArrived=on
      | getData(entity.Data);
      | %calcDelay(entity.Time);
      settings: OutputPortMap=o0
  TX Message : EntityMulticast  InputPortMessageModes=m  MulticastTag=ToBus_2
  Transmission Buffer : EntityQueue  InputPortMessageModes=m  OutputPortMessageModes=n,m  Capacity=15  QueueType=Priority  PrioritySource=ID  NumberEntitiesInBlock=on
      settings: OutputPortMap=o1,o5
  Unsubscribed Message : EntityTerminator  InputPortMessageModes=m  NumberEntitiesArrived=on
      settings: OutputPortMap=o0
  Entity_received : Outport
  wires:
  Replicate for Re-Transmission1/1 -> Subscribed Message/1
  Replicate for Re-Transmission1/2 -> Entity_received/1
  Subscribed Message/1 -> Scope2/1
  Replicate for Re-Transmission2/2 -> Entity Terminator2/1
  Replicate for Re-Transmission2/1 -> TX Message/1
  Simulink Function1/1(data) -> Scope11/1
  RX Takt/1(Out) -> Entity Replicator/1
  Path Combiner/1 -> Transmission Buffer/1
  Drop Dated Message upon Buffer Overflow/2 -> Entity Terminator/1
  Simulink Function2/1(ctrl) -> Re-Transmission Control/1(Msg_available)
  Entity Terminator/1 -> Scope10/1
  ACK Message/1 -> Scope12/1
  Entity Replicator/1 -> Reception Control/3(RX)
  Entity_transmit/1 -> Path Combiner/2
  Sort/1 -> Replicate for Re-Transmission1/1
  RX Message/1 -> Scope7/1
  Re-Transmission Control/2(#TX) -> #TX/1
  Drop Dated Message upon Buffer Overflow/1 -> Path Combiner/1
  Current Message/1 -> Re-Transmission Control/4(IN)
  Entity Terminator2/1 -> Scope1/1
  Entity Replicator/3 -> Damaged Message1/1
  Damaged Message1/1 -> Scope6/1
  Reception Control/3(ReTX) -> [ReTX]
  [ReTX] -> Re-Transmission Control/2(ReTX)
  Received Message/1 -> Sort/2
  Transmission Buffer/2 -> Message Release Control/2
  Message Release Control/1 -> Replicate for Re-Transmission/1
  Replicate for Re-Transmission/1 -> Current Message/1
  [Reset] -> Re-Transmission Control/3(Reset)
  Sort/2 -> Unsubscribed Message/1
  Sort/3 -> Damaged Message/1
  Entity Replicator/2 -> Received Message/1
  Reception Control/2(Success) -> [Reset]
  Reception Control/1(Port) -> Sort/1
  Replicate for Re-Transmission/3 -> Reception Control/1(TX)
  Simulink Function/1(ctrl) -> Message Release Control/1
  Replicate for Re-Transmission/2 -> Replicate for Re-Transmission2/1
  Re-Transmission Control/1(OUT) -> Drop Dated Message upon Buffer Overflow/1
  Unsubscribed Message/1 -> Scope4/1
  Damaged Message/1 -> Scope5/1
  Transmission Buffer/1 -> Scope8/1
  ACK Takt/1(Out) -> Reception Control/2(ACK)
  ACK Message/2 -> ACK Takt/1(In)
  RX Message/2 -> RX Takt/1(In)

== system NCS_Library/Network/CAN/Logik ==
  In_fast : Inport
  In_slow : Inport  Port=2
  Fast_to_Slow : Subsystem
  Resource Pool : EntityResourcePool  ResourceName=Token1  ResourceAmount=1  AmountInUse=on
  Scope43 : Scope
  Slow_to_Fast : Subsystem
  Out_slow : Outport
  Out_fast : Outport  Port=2
  wires:
  Fast_to_Slow/1(Out) -> Out_slow/1
  Slow_to_Fast/1(Out) -> Out_fast/1
  In_slow/1 -> Slow_to_Fast/1(In)
  In_fast/1 -> Fast_to_Slow/1(In)
  Resource Pool/1 -> Scope43/1

== system NCS_Library/Network/ETB/Burst Device ==
  note: User defined Parameters
  RxFromBus : Inport
  Add : Sum  Inputs=+-
  Bus Creator : BusCreator  Inputs=8
  Constant : Constant  Value=Address  OutDataTypeStr=uint16
  Constant1 : Constant  Value=Destination  OutDataTypeStr=uint16
  Constant2 : Constant  Value=Tx  OutDataTypeStr=double
  Constant3 : Constant  Value=msgType  OutDataTypeStr=uint8
  Constant4 : Constant  Value=SDTv2  OutDataTypeStr=double
  Constant5 : Constant
  Constant6 : Constant  Value=Port  OutDataTypeStr=uint16
  Constant7 : Constant  Value=ReplyAddress  OutDataTypeStr=uint16
  Constant8 : Constant  Value=zeros(3,20)
  Display : Display
  Entity Gate : EntityGate  InputPortMessageModes=m,m  OutputPortMessageModes=m
  Entity Queue : EntityQueue  InputPortMessageModes=m  OutputPortMessageModes=n,m  Capacity=n_Burst  NumberEntitiesInBlock=on
      settings: OutputPortMap=o1,o5
  Failure Control : $bdroot/Network/Applications/Failure Control  SystemSampleTime=-1
  Failure Control1 : $bdroot/Network/Applications/Failure Control  SystemSampleTime=-1
  MATLAB Function : MATLAB Function  TreatAsAtomicUnit=on
  MATLAB Function1 : MATLAB Function  TreatAsAtomicUnit=on
  Message Send : MessageSend  OutputPortMessageModes=m
      settings: InputPortMap=u1
  Protocl Stack : Subsystem
  Subscribe : Constant  Value=Subscribe  OutDataTypeStr=uint16
  Subsystem : Subsystem
  Subsystem1 : Subsystem
  Subsystem2 : Subsystem
  Subsystem3 : Subsystem
  Subsystem4 : $bdroot/Network/Applications/Subsystem  SystemSampleTime=-1
  Terminator : Terminator
  Terminator1 : Terminator
  TxToBus : Outport
  wires:
  Failure Control/1 -> Protocl Stack/3(RxFromBus)
  MATLAB Function1/1(y) -> Bus Creator/3  "Subscribe"
  Protocl Stack/3(TxToBus) -> Failure Control1/1
  RxFromBus/1 -> Failure Control/1
  Subsystem3/1(Out1) -> Bus Creator/4  "ReplyAddress"
  Subsystem2/1(Out1) -> Bus Creator/2  "Destination"
  Subsystem1/1(Out1) -> Bus Creator/1  "Address"
  Constant7/1 -> Subsystem3/1(In1)
  Constant6/1 -> Bus Creator/5  "Port"
  Subscribe/1 -> MATLAB Function1/1(u)
  Constant2/1 -> Bus Creator/6  "T_Tx"
  Constant1/1 -> Subsystem2/1(In1)
  Constant/1 -> Subsystem1/1(In1)
  Bus Creator/1 -> Protocl Stack/2(Parameter)
  Protocl Stack/1(Data) -> Terminator/1
  Protocl Stack/2(Recorder) -> Terminator1/1
  MATLAB Function/1(msgType) -> Bus Creator/7  "msgType"
  Constant3/1 -> MATLAB Function/1(u)
  Add/1 -> Bus Creator/8  "SDTv2"
  Constant4/1 -> Add/1
  Constant5/1 -> Add/2
  Constant8/1 -> Protocl Stack/1(Signal)
  Entity Gate/1 -> TxToBus/1
  Entity Queue/2 -> Entity Gate/2
  Entity Queue/1 -> Display/1
  Failure Control1/1 -> Subsystem/1(In1)
  Message Send/1 -> Entity Gate/1
  Subsystem4/1 -> Message Send/1
  Subsystem/1(Out1) -> Entity Queue/1

== system NCS_Library/Network/ETB/Cable ==
  IN_R : Inport
  IN_L : Inport  Port=2
  Cable Length : Constant  Value=length
  Clock : Clock
  Constant : Constant  Value=Cable
  Display : Display
  Display1 : Display
  Display2 : Display
  Entity Server : EntityServer  InputPortMessageModes=n,m  OutputPortMessageModes=n,m  Capacity=inf  ServiceTimeSource=Signal port  ServiceTimeValue=CableLength/3e8  EntryAction=entity.CheckBit = BitError(entity.Source, entity.SEQ);  NumberEntitiesDeparted=on
      settings: InputPortMap=u0,u2  OutputPortMap=o0,o9
  Entity Server1 : EntityServer  InputPortMessageModes=n,m  OutputPortMessageModes=n,m  Capacity=inf  ServiceTimeSource=Signal port  ServiceTimeValue=CableLength/3e8  EntryAction=entity.CheckBit = BitError(entity.Source, entity.SEQ);  NumberEntitiesDeparted=on
      settings: InputPortMap=u0,u2  OutputPortMap=o0,o9
  MATLAB Function : MATLAB Function  TreatAsAtomicUnit=on
  Product of Elements : Product  Inputs=*//
  Simulink Function : Subsystem  TreatAsAtomicUnit=on
  Speed of light : Constant  Value=3e8
  OUT_L : Outport
  OUT_R : Outport  Port=2
  wires:
  Entity Server/2 -> OUT_R/1
  Entity Server1/2 -> OUT_L/1
  IN_L/1 -> Entity Server/2
  IN_R/1 -> Entity Server1/2
  Product of Elements/1 -> Entity Server1/1, Entity Server/1  "Delta_t"
  Entity Server/1 -> Display/1
  Clock/1 -> Simulink Function/1(Time)
  Speed of light/1 -> Product of Elements/3  "c"
  Cable Length/1 -> Product of Elements/1
  MATLAB Function/1(NVP) -> Display1/1, Product of Elements/2  "NVP"
  Constant/1 -> MATLAB Function/1(Cable)
  Entity Server1/1 -> Display2/1
